simulink model "VDCHyd2020a"  (R2020a)
settings: Solver=daessc  StartTime=0.0  StopTime=simulationEndTime  FixedStep=0.001  RelTol=1e-2
values from neighbouring files (symbols this model uses):
  Bc1_V = [0;0;0;0;0;0]    [initializeSimulationGP.m]
  filtDV = init2ndOrderLowPassFilter(35*2*pi,1,controller.dT)    [initializeLowPassFilters.m]
  filtEnc = init2ndOrderLowPassFilter(35*2*pi,1,controller.dT)    [initializeLowPassFilters.m]
undefined symbols (not defined in the file or in its folder): aux, B11_r_B11Tc1, B11_V, B11_Vr, B11Ftot_r, B12_r_B12Tc2, B12_Rot_Tc2, B12_U_Tc2, B12_V, B12_Vr, B12Ftot_r, B31_r_B31B41, B31_V, B31_Vr, B31FTot_r, B32_r_B32B42, B32_Rot_B42, B32_U_B42, B32_V, B32_Vr, B32FTot_r, B41_r_B41Tc1, B41_V, B41_Vr, B41FTot_r, B42_r_B42Tc2, B42_Rot_Tc2, B42_U_Tc2, B42_V, B42_Vr, B42FTot_r, B52_r_B52P32, B52_Rot_P32, B52_U_P32, B52_V, B52_Vr, B52Ftot_r, Bc1_r_Bc1B11, Bc1_r_Bc1B31, Bc1_Vr, Bc1FTot_r, Bc2_r_Bc2B12, Bc2_r_Bc2B32, Bc2_Rot_B12, Bc2_Rot_B32, Bc2_U_B12, Bc2_U_B32, Bc2_V, Bc2_Vr, Bc2Tot_r, controller, cyl1, cyl2, cylT2, D22_V, D22_Vr, D22Fr, DiscIntNeverNeededParam, dq1, dq11 ... (+125)
libraries: sm_lib x34, nesl_utility x15, simulink x11, dspinverses x1
(part 3 of 12)

== system VDCHyd2020a/sbHydraulicManipulatorSimscape/sbTilitLink ==
  P22p_to_P22 : sm_lib/Frames and Transforms/Rigid Transform  TranslationMethod=StandardAxis  TranslationStandardOffset=17  TranslationLengthUnit=mm  TranslationStandardAxis=+Z  TranslationCartesianOffset=[0 0 0]  TranslationROffset=0  TranslationROffsetUnits=m  TranslationZOffset=0  TranslationZOffsetUnits=m  TranslationThetaOffset=0  TranslationThetaOffsetUnits=deg  RotationMethod=None  RotationAngleUnits=deg  RotationStandardAxis=+Z  RotationAngle=0.0  RotationArbitraryAxis=[0 0 1]  FollAlignAxisA=+X  BaseAlignAxisA=+Y  FollAlignAxisB=+Y  BaseAlignAxisB=+Z  RotationSequenceAxes=FollowerAxes  RotationSequence=XYX  RotationSequenceAngles=[0 0 0]  RotationSequenceAnglesUnits=deg  RotationMatrix=[1 0 0; 0 1 0; 0 0 1]
  TiltLinkSolid : sm_lib/Body Elements/File Solid  ExtGeomFileName=07_TiltLinkGP.STEP  UnitType=Custom  ExtGeomFileUnits=m  StepReaderType=OCC  ExportConvexHullGeometry=off  InertiaType=Custom  Mass=33.92850233  MassUnits=kg  CenterOfMass=[0.53783811 -0.04670816 0.00002484]  CenterOfMassUnits=m  MomentsOfInertia=[0.31079192 7.19217974 7.40915161]  MomentsOfInertiaUnits=kg*m^2  ProductsOfInertia=[-0.00058487 0.00275052 -0.58280922]  ProductsOfInertiaUnits=kg*m^2  BasedOnType=Density  Density=7300  DensityUnits=kg/m^3  DoExposeReferenceFrame=off  SerializedFrames=<Frames><Frame><Id>Frame1</Id><Value><Name>F5rot</Name><Origin><Source>GeometricFeature</Source><FeatureName>cylindrical surface 12</FeatureName></Origin><PrimaryAxis><DefinedDirection>+Z</DefinedDirection><Source>ReferenceFrame</Source><SourceDirection>+Z</SourceDirection><FeatureName></FeatureName></PrimaryAxis><SecondaryAxis><DefinedDirection>+X</DefinedDirection><Source>ReferenceFrame</Source><SourceDirection>+X</SourceDirection><FeatureName></FeatureName></SecondaryAxis></Value></Frame><Frame><Id>Frame2</Id><Value><Name>F6</Name><Origin><Source>GeometricFeature</Source><FeatureName>cylindrical surface 13</FeatureName></Origin><PrimaryAxis><DefinedDirection>+Z</DefinedDirection><Source>ReferenceFrame</Source><SourceDirection>+Z</SourceDirection><FeatureName></FeatureName></PrimaryAxis><SecondaryAxis><DefinedDirection>+X</DefinedDirection><Source>ReferenceFrame</Source><SourceDirection>+X</SourceDirection><FeatureName></FeatureName></SecondaryAxis></Value></Frame><Frame><Id>Frame3</Id><Value><Name>P22p</Name><Origin><Source>GeometricFeature</Source><FeatureName>circular curve 59</FeatureName></Origin><PrimaryAxis><DefinedDirection>+Y</DefinedDirection><Source>GeometricFeature</Source><SourceDirection>+Z</SourceDirection><FeatureName>segment 349</FeatureName></PrimaryAxis><SecondaryAxis><DefinedDirection>+X</DefinedDirection><Source>ReferenceFrame</Source><SourceDirection>+X</SourceDirection><FeatureName></FeatureName></SecondaryAxis></Value></Frame><Frame><Id>Frame4</Id><Value><Name>Tc2p</Name><Origin><Source>GeometricFeature</Source><FeatureName>cylindrical surface 13</FeatureName></Origin><PrimaryAxis><DefinedDirection>+X</DefinedDirection><Source>GeometricFeature</Source><SourceDirection>+Z</SourceDirection><FeatureName>segment 205</FeatureName></PrimaryAxis><SecondaryAxis><DefinedDirection>+Y</DefinedDirection><Source>ReferenceFrame</Source><SourceDirection>+X</SourceDirection><FeatureName></FeatureName></SecondaryAxis></Value></Frame><Frame><Id>Frame5</Id><Value><Name>B12</Name><Origin><Source>GeometricFeature</Source><FeatureName>cylindrical surface 12</FeatureName></Origin><PrimaryAxis><DefinedDirection>-X</DefinedDirection><Source>GeometricFeature</Source><SourceDirection>+Z</SourceDirection><FeatureName>segment 203</FeatureName></PrimaryAxis><SecondaryAxis><DefinedDirection>+Y</DefinedDirection><Source>ReferenceFrame</Source><SourceDirection>+X</SourceDirection><FeatureName></FeatureName></SecondaryAxis></Value></Frame></Frames>  GraphicType=FromGeometry  MarkerShape=Sphere  MarkerSize=10  GraphicVisPropType=SimpleVisualProperties  GraphicDiffuseColor=[134 134 255]/255  GraphicSpecularColor=[0.5 0.5 0.5 1.0]  GraphicAmbientColor=[0.15 0.15 0.15 1.0]  GraphicEmissiveColor=[0.0 0.0 0.0 1.0]  GraphicShininess=75  GraphicOpacity=1.0
  P22 : PMIOPort  Side=Left
  Tc2 : PMIOPort  Port=2  Side=Left
  B12 : PMIOPort  Port=3  Side=Left
  F6 : PMIOPort  Port=4  Side=Left
  F5_rot : PMIOPort  Port=5  Side=Right
  connections:
  F5_rot/RConn1 -- TiltLinkSolid/LConn1
  F6/RConn1 -- TiltLinkSolid/RConn1
  P22p_to_P22/RConn1 -- P22/RConn1
  P22p_to_P22/LConn1 -- TiltLinkSolid/LConn2
  Tc2/RConn1 -- TiltLinkSolid/RConn2
  B12/RConn1 -- TiltLinkSolid/LConn3

== system VDCHyd2020a/sbHydraulicManipulatorSimscape/sbTiltCylinderAndTiltPiston ==
  note: Friction force...
  fp2 : Inport
  B32Aux : sm_lib/Frames and Transforms/Rigid Transform  TranslationMethod=None  TranslationStandardOffset=0  TranslationLengthUnit=m  TranslationStandardAxis=+Z  TranslationCartesianOffset=[0 0 0]  TranslationROffset=0  TranslationROffsetUnits=m  TranslationZOffset=0  TranslationZOffsetUnits=m  TranslationThetaOffset=0  TranslationThetaOffsetUnits=deg  RotationMethod=StandardAxis  RotationAngleUnits=deg  RotationStandardAxis=+Y  RotationAngle=90  RotationArbitraryAxis=[0 0 1]  FollAlignAxisA=+X  BaseAlignAxisA=+Y  FollAlignAxisB=+Y  BaseAlignAxisB=+Z  RotationSequenceAxes=FollowerAxes  RotationSequence=XYX  RotationSequenceAngles=[0 0 0]  RotationSequenceAnglesUnits=deg  RotationMatrix=[1 0 0; 0 1 0; 0 0 1]
  B42Aux : sm_lib/Frames and Transforms/Rigid Transform  TranslationMethod=None  TranslationStandardOffset=0  TranslationLengthUnit=m  TranslationStandardAxis=+Z  TranslationCartesianOffset=[0 0 0]  TranslationROffset=0  TranslationROffsetUnits=m  TranslationZOffset=0  TranslationZOffsetUnits=m  TranslationThetaOffset=0  TranslationThetaOffsetUnits=deg  RotationMethod=StandardAxis  RotationAngleUnits=deg  RotationStandardAxis=+Y  RotationAngle=-90  RotationArbitraryAxis=[0 0 1]  FollAlignAxisA=+X  BaseAlignAxisA=+Y  FollAlignAxisB=+Y  BaseAlignAxisB=+Z  RotationSequenceAxes=FollowerAxes  RotationSequence=XYX  RotationSequenceAngles=[0 0 0]  RotationSequenceAnglesUnits=deg  RotationMatrix=[1 0 0; 0 1 0; 0 0 1]
  Constant : Constant  Value=settings.actuatorFrictionON
  Constant1 : Constant  Value=0
  PS-Sim1 : nesl_utility/PS-Simulink Converter  PhysicalDomain=network_engine_domain  SubClassName=ps_output  LeftPortType=input  RightPortType=output  PseudoPeriodic=off  Frequencies=[]  VectorFormat=1-D array  Unit=inherit  AffineConversion=off
      settings: SourceProductBaseCode=SS,PW,VE
  PS-Sim2 : nesl_utility/PS-Simulink Converter  PhysicalDomain=network_engine_domain  SubClassName=ps_output  LeftPortType=input  RightPortType=output  PseudoPeriodic=off  Frequencies=[]  VectorFormat=1-D array  Unit=inherit  AffineConversion=off
      settings: SourceProductBaseCode=SS,PW,VE
  Simulink-PS Converter : nesl_utility/Simulink-PS Converter  PhysicalDomain=network_engine_domain  SubClassName=ps_input  LeftPortType=input  RightPortType=output  PseudoPeriodic=off  Frequencies=[]  NoiseDistribution=none  NoiseParameters=[]  Unit=1  AffineConversion=off  FilteringAndDerivatives=provide  SimscapeFilterOrder=1  InputFilterTimeConstant=0.001  UdotUserProvided=0
      settings: SourceProductBaseCode=SS,PW,VE
  Sum : Sum  Inputs=|+-
  Switch : Switch  Criteria=u2 > Threshold
  TiltCylinderSolid : sm_lib/Body Elements/File Solid  ExtGeomFileName=05_TiltCylGP.STEP  UnitType=FromFile  ExtGeomFileUnits=m  StepReaderType=OCC  ExportConvexHullGeometry=off  InertiaType=Custom  Mass=17.36281648  MassUnits=kg  CenterOfMass=[0 0.31781210 0]  CenterOfMassUnits=m  MomentsOfInertia=[0.90735702 0.03150902 0.90763033]  MomentsOfInertiaUnits=kg*m^2  ProductsOfInertia=[0 0 0]  ProductsOfInertiaUnits=kg*m^2  BasedOnType=Density  Density=7300  DensityUnits=kg/m^3  DoExposeReferenceFrame=off  SerializedFrames=<Frames><Frame><Id>Frame1</Id><Value><Name>B32</Name><Origin><Source>GeometricFeature</Source><FeatureName>cylindrical surface 11</FeatureName></Origin><PrimaryAxis><DefinedDirection>+X</DefinedDirection><Source>ReferenceFrame</Source><SourceDirection>+Y</SourceDirection><FeatureName></FeatureName></PrimaryAxis><SecondaryAxis><DefinedDirection>+Y</DefinedDirection><Source>ReferenceFrame</Source><SourceDirection>-X</SourceDirection><FeatureName></FeatureName></SecondaryAxis></Value></Frame><Frame><Id>Frame2</Id><Value><Name>B32Aux</Name><Origin><Source>GeometricFeature</Source><FeatureName>planar surface 4</FeatureName></Origin><PrimaryAxis><DefinedDirection>+X</DefinedDirection><Source>ReferenceFrame</Source><SourceDirection>+Y</SourceDirection><FeatureName></FeatureName></PrimaryAxis><SecondaryAxis><DefinedDirection>+Y</DefinedDirection><Source>ReferenceFrame</Source><SourceDirection>-X</SourceDirection><FeatureName></FeatureName></SecondaryAxis></Value></Frame></Frames>  GraphicType=FromGeometry  MarkerShape=Sphere  MarkerSize=10  GraphicVisPropType=SimpleVisualProperties  GraphicDiffuseColor=[1 1 119]/255  GraphicSpecularColor=[0.5 0.5 0.5 1.0]  GraphicAmbientColor=[0.15 0.15 0.15 1.0]  GraphicEmissiveColor=[0.0 0.0 0.0 1.0]  GraphicShininess=75  GraphicOpacity=1.0
  TiltPistonSolid : sm_lib/Body Elements/File Solid  ExtGeomFileName=06_TiltPistGP.STEP  UnitType=FromFile  ExtGeomFileUnits=m  StepReaderType=OCC  ExportConvexHullGeometry=off  InertiaType=Custom  Mass=10.34519231  MassUnits=kg  CenterOfMass=[0 0.32981882 0]  CenterOfMassUnits=m  MomentsOfInertia=[0.55759812 0.00370720 0.55785997]  MomentsOfInertiaUnits=kg*m^2  ProductsOfInertia=[0 0 0]  ProductsOfInertiaUnits=kg*m^2  BasedOnType=Density  Density=7850  DensityUnits=kg/m^3  DoExposeReferenceFrame=off  SerializedFrames=<Frames><Frame><Id>Frame2</Id><Value><Name>B42</Name><Origin><Source>GeometricFeature</Source><FeatureName>planar surface 2</FeatureName></Origin><PrimaryAxis><DefinedDirection>+X</DefinedDirection><Source>ReferenceFrame</Source><SourceDirection>+Y</SourceDirection><FeatureName></FeatureName></PrimaryAxis><SecondaryAxis><DefinedDirection>+Y</DefinedDirection><Source>ReferenceFrame</Source><SourceDirection>-X</SourceDirection><FeatureName></FeatureName></SecondaryAxis></Value></Frame><Frame><Id>Frame3</Id><Value><Name>P11</Name><Origin><Source>GeometricFeature</Source><FeatureName>cylindrical surface 8</FeatureName></Origin><PrimaryAxis><DefinedDirection>+X</DefinedDirection><Source>ReferenceFrame</Source><SourceDirection>+Y</SourceDirection><FeatureName></FeatureName></PrimaryAxis><SecondaryAxis><DefinedDirection>+Y</DefinedDirection><Source>ReferenceFrame</Source><SourceDirection>-X</SourceDirection><FeatureName></FeatureName></SecondaryAxis></Value></Frame></Frames>  GraphicType=FromGeometry  MarkerShape=Sphere  MarkerSize=10  GraphicVisPropType=SimpleVisualProperties  GraphicDiffuseColor=[9 232 232]/255  GraphicSpecularColor=[0.5 0.5 0.5 1.0]  GraphicAmbientColor=[0.15 0.15 0.15 1.0]  GraphicEmissiveColor=[0.0 0.0 0.0 1.0]  GraphicShininess=75  GraphicOpacity=1.0
  q21Rotation : sm_lib/Joints/Revolute Joint  JointMode=Normal  SenseConstraintForce=off  SenseConstraintForceX=off  SenseConstraintForceY=off  SenseConstraintForceZ=off  SenseConstraintTorque=off  SenseConstraintTorqueX=off  SenseConstraintTorqueY=off  SenseConstraintTorqueZ=off  SenseTotalForce=off  SenseTotalForceX=off  SenseTotalForceY=off  SenseTotalForceZ=off  SenseTotalTorque=off  SenseTotalTorqueX=off  SenseTotalTorqueY=off  SenseTotalTorqueZ=off  CompositeWrenchDir=FollowerOnBase  CompositeWrenchFrame=BaseFrame  EquilibriumPosition=0  EquilibriumPositionUnits=rad  SpringStiffness=0  SpringStiffnessUnits=N*m/rad  DampingCoefficient=revJoint2.damp  DampingCoefficientUnits=N*m/(rad/s)  TorqueActuationMode=NoTorque  MotionActuationMode=ComputedMotion  SensePosition=off  SenseVelocity=off  SenseAcceleration=off  SenseTorqueForce=off  SenseLowerLimitTorqueForce=off  SenseUpperLimitTorqueForce=off  LowerLimitSpecify=off  LowerLimitBound=-90  LowerLimitBoundUnits=deg  LowerLimitStiffness=1e4  LowerLimitStiffnessUnits=N*m/deg  LowerLimitDamping=10  LowerLimitDampingUnits=N*m/(deg/s)  LowerLimitTransitionRegionWidth=0.1  LowerLimitTransitionRegionWidthUnits=deg  UpperLimitSpecify=off  UpperLimitBound=90  UpperLimitBoundUnits=deg  UpperLimitStiffness=1e4  UpperLimitStiffnessUnits=N*m/deg  UpperLimitDamping=10  UpperLimitDampingUnits=N*m/(deg/s)  UpperLimitTransitionRegionWidth=0.1  UpperLimitTransitionRegionWidthUnits=deg  PositionTargetSpecify=off  PositionTargetPriority=High  PositionTargetValue=0  PositionTargetValueUnits=deg  VelocityTargetSpecify=off  VelocityTargetPriority=High  VelocityTargetValue=0  VelocityTargetValueUnits=deg/s
  q22Rotation : sm_lib/Joints/Revolute Joint  JointMode=Normal  SenseConstraintForce=off  SenseConstraintForceX=off  SenseConstraintForceY=off  SenseConstraintForceZ=off  SenseConstraintTorque=off  SenseConstraintTorqueX=off  SenseConstraintTorqueY=off  SenseConstraintTorqueZ=off  SenseTotalForce=off  SenseTotalForceX=off  SenseTotalForceY=off  SenseTotalForceZ=off  SenseTotalTorque=off  SenseTotalTorqueX=off  SenseTotalTorqueY=off  SenseTotalTorqueZ=off  CompositeWrenchDir=FollowerOnBase  CompositeWrenchFrame=BaseFrame  EquilibriumPosition=0  EquilibriumPositionUnits=rad  SpringStiffness=0  SpringStiffnessUnits=N*m/rad  DampingCoefficient=revJoint2.damp  DampingCoefficientUnits=N*m/(rad/s)  TorqueActuationMode=NoTorque  MotionActuationMode=ComputedMotion  SensePosition=off  SenseVelocity=off  SenseAcceleration=off  SenseTorqueForce=off  SenseLowerLimitTorqueForce=off  SenseUpperLimitTorqueForce=off  LowerLimitSpecify=off  LowerLimitBound=-90  LowerLimitBoundUnits=deg  LowerLimitStiffness=1e4  LowerLimitStiffnessUnits=N*m/deg  LowerLimitDamping=10  LowerLimitDampingUnits=N*m/(deg/s)  LowerLimitTransitionRegionWidth=0.1  LowerLimitTransitionRegionWidthUnits=deg  UpperLimitSpecify=off  UpperLimitBound=90  UpperLimitBoundUnits=deg  UpperLimitStiffness=1e4  UpperLimitStiffnessUnits=N*m/deg  UpperLimitDamping=10  UpperLimitDampingUnits=N*m/(deg/s)  UpperLimitTransitionRegionWidth=0.1  UpperLimitTransitionRegionWidthUnits=deg  PositionTargetSpecify=off  PositionTargetPriority=High  PositionTargetValue=0  PositionTargetValueUnits=deg  VelocityTargetSpecify=off  VelocityTargetPriority=High  VelocityTargetValue=0  VelocityTargetValueUnits=deg/s
  sbFrictionForceRS2 : Subsystem
  x2-translation : sm_lib/Joints/Prismatic Joint  JointMode=Normal  SenseConstraintForce=off  SenseConstraintForceX=off  SenseConstraintForceY=off  SenseConstraintForceZ=off  SenseConstraintTorque=off  SenseConstraintTorqueX=off  SenseConstraintTorqueY=off  SenseConstraintTorqueZ=off  SenseTotalForce=off  SenseTotalForceX=off  SenseTotalForceY=off  SenseTotalForceZ=off  SenseTotalTorque=off  SenseTotalTorqueX=off  SenseTotalTorqueY=off  SenseTotalTorqueZ=off  CompositeWrenchDir=FollowerOnBase  CompositeWrenchFrame=FollowerFrame  EquilibriumPosition=0  EquilibriumPositionUnits=m  SpringStiffness=0  SpringStiffnessUnits=N/m  DampingCoefficient=0  DampingCoefficientUnits=N/(m/s)  TorqueActuationMode=InputTorque  MotionActuationMode=ComputedMotion  SensePosition=on  SenseVelocity=on  SenseAcceleration=off  SenseTorqueForce=off  SenseLowerLimitTorqueForce=off  SenseUpperLimitTorqueForce=off  LowerLimitSpecify=on  LowerLimitBound=0  LowerLimitBoundUnits=m  LowerLimitStiffness=1e6  LowerLimitStiffnessUnits=N/m  LowerLimitDamping=1e3  LowerLimitDampingUnits=N/(m/s)  LowerLimitTransitionRegionWidth=1e-4  LowerLimitTransitionRegionWidthUnits=m  UpperLimitSpecify=on  UpperLimitBound=cyl2.sp  UpperLimitBoundUnits=m  UpperLimitStiffness=1e6  UpperLimitStiffnessUnits=N/m  UpperLimitDamping=1e3  UpperLimitDampingUnits=N/(m/s)  UpperLimitTransitionRegionWidth=1e-4  UpperLimitTransitionRegionWidthUnits=m  PositionTargetSpecify=on  PositionTargetPriority=Low  PositionTargetValue=0.3  PositionTargetValueUnits=m  VelocityTargetSpecify=on  VelocityTargetPriority=High  VelocityTargetValue=0  VelocityTargetValueUnits=m/s
  B32 : PMIOPort  Side=Left
  B42 : PMIOPort  Port=2  Side=Left
  F4 : PMIOPort  Port=3  Side=Right
  F6 : PMIOPort  Port=4  Side=Right
  x2 : Outport
  dx2 : Outport  Port=2
  wires:
  PS-Sim2/1 -> x2/1
  fp2/1 -> sbFrictionForceRS2/2(fp2), Sum/1
  Sum/1 -> Simulink-PS Converter/1
  Switch/1 -> Sum/2
  PS-Sim1/1 -> sbFrictionForceRS2/1(dx2), dx2/1
  sbFrictionForceRS2/1(ff2) -> Switch/1
  Constant1/1 -> Switch/3
  Constant/1 -> Switch/2
  connections:
  TiltCylinderSolid/RConn1 -- B32Aux/LConn1
  x2-translation/RConn1 -- B42Aux/LConn1
  q21Rotation/RConn1 -- TiltCylinderSolid/LConn1 -- B32/RConn1
  B42/RConn1 -- TiltPistonSolid/LConn1 -- B42Aux/RConn1
  B32Aux/RConn1 -- x2-translation/LConn1
  q21Rotation/LConn1 -- F4/RConn1
  TiltPistonSolid/RConn1 -- q22Rotation/LConn1
  q22Rotation/RConn1 -- F6/RConn1
  x2-translation/RConn2 -- PS-Sim2/LConn1
  Simulink-PS Converter/RConn1 -- x2-translation/LConn2
  PS-Sim1/LConn1 -- x2-translation/RConn3

== system VDCHyd2020a/sbVDCController/sbAuxiliaryJointAngles ==
  note: For more details on relations in this subsystem, please see the supplementary pdf at:
      | https://se.mathworks.com/matlabcentral/fileexchange/123465-calculating-actuator-forces-on-a-hardware-target
      |
      | In the paper qj angles are assumed known beforehand...
  note: Calculate q1 and q2 from measured Theta1 and Theta2 angles...
  note: Get inputs...
  note: Process data...
  note: Pass to outputs...
  theta1Filt : Inport
  theta2Filt : Inport  Port=2
  q1Angle : MATLAB Function  TreatAsAtomicUnit=on
  q2Angle : MATLAB Function  TreatAsAtomicUnit=on
  q1 : Outport
  q2 : Outport  Port=2
  wires:
  q2Angle/1(q2) -> [q2]  "q2"
  [q2] -> q2/1  "q2"
  [q1] -> q1/1  "q1"
  q1Angle/1(q1) -> [q1]  "q1"
  [theta1Filt] -> q1Angle/1(theta1)  "theta1Filt"
  [theta2Filt] -> q2Angle/1(theta2)  "theta2Filt"
  theta2Filt/1 -> [theta2Filt]  "theta2Filt"
  theta1Filt/1 -> [theta1Filt]  "theta1Filt"

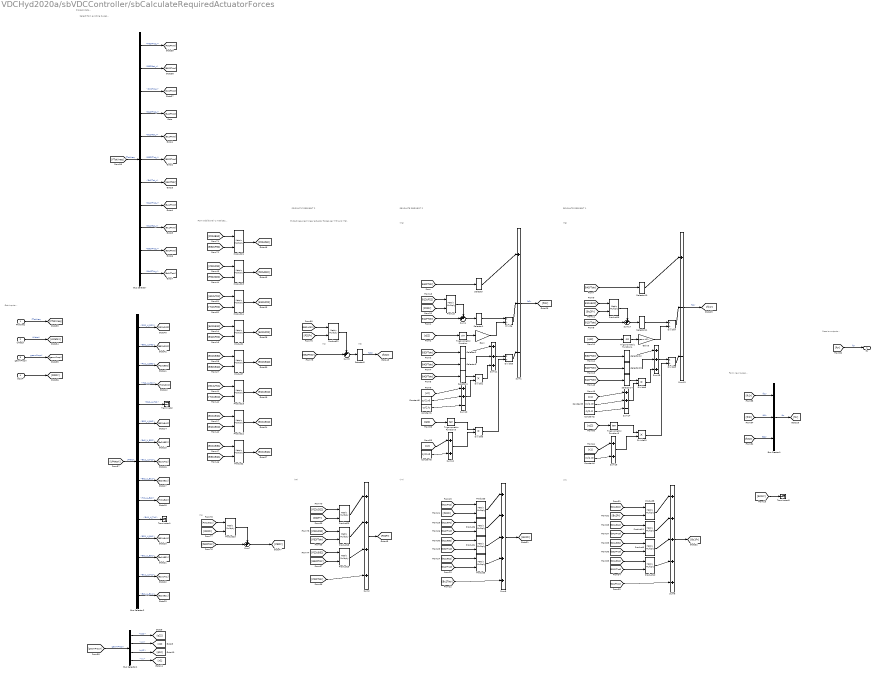
== system VDCHyd2020a/sbVDCController/sbCalculateRequiredActuatorForces ==
  note: (73)
  note: Get inputs...
  note: Select from existing buses...
  note: Form additional U matrices...
  note: (76)
  note: (76)
  note: (77)
  note: (77)
  note: Extract required linear actuator forces per (73) and (76).
  note: Process data...
  note: Form new buses...
  note: Pass to outputs...
  note: (74)
  note: (71)
  note: (72)
  note: REVOLUTE SEGMENT 2
  note: REVOLUTE SEGMENT 1
  note: PRISMATIC SEGMENT 2
  FTotXreq : Inport
  UMatsX : Inport  Port=2
  geomPropX : Inport  Port=3
  D22Fr : Inport  Port=4
  Bus Creator1 : BusCreator  Inputs=fc1r,fc2r,fct2r
  Bus Selector : BusSelector  OutputSignals=FTotPS2req.P32FTot_r,FTotPS2req.B52Ftot_r,FTotPS2req.P22Tot_r,FTotRS2req.B42FTot_r,FTotRS2req.B12Ftot_r,FTotRS2req.B32FTot_r,FTotRS2req.Bc2Tot_r,FTotRS1req.B41FTot_r,FTotRS1req.B11Ftot_r,FTotRS1req.B31FTot_r,FTotRS1req.Bc1FTot_r
  Bus Selector1 : BusSelector  OutputSignals=geomPropRS2.q22,geomPropRS2.x2,geomPropRS1.q12,geomPropRS1.x1
  Bus Selector2 : BusSelector  OutputSignals=UMatsPS2.P32_U_D22,UMatsPS2.B52_U_P32,UMatsPS2.P22_U_B52,UMatsRS2.Tc2_U_P22,UMatsRS2.B42_U_Tc2,UMatsRS2.B32_U_B42,UMatsRS2.Bc2_U_B32,UMatsRS2.B12_U_Tc2,UMatsRS2.Bc2_U_B12,UMatsRS1.Tc1_U_Bc2,UMatsRS1.B41_U_Tc1,UMatsRS1.B31_U_B41,UMatsRS1.Bc1_U_B31,UMatsRS1.B11_U_Tc1,UMatsRS1.Bc1_U_B11
  Constant1 : Constant  Value=cyl2.lc
  Constant2 : Constant  Value=cyl1.lc
  Constant3 : Constant  Value=cyl1.x0
  Constant4 : Constant  Value=cyl1.x0
  Constant5 : Constant  Value=cyl2.x0
  Constant6 : Constant  Value=cyl2.x0
  Divide{,5,7,9} (4 alike) : Product  Inputs=*/
  Divide{1,6,8,10} (4 alike) : Product  Inputs=**
  Gain : Gain  Gain=geom.L21
  Gain5 : Gain  Gain=geom.L11
  Product{,1..16,18..23} (23 alike) : Product  Multiplication=Matrix(*)
  Selector : Selector  IndexMode=Zero-based  InputPortWidth=6  IndexOptions=Index vector (dialog)  Indices=[0]  OutputSizes=1
  Selector{1..3,11..13} (6 alike) : Selector  IndexMode=Zero-based  InputPortWidth=6  IndexOptions=Index vector (dialog)  Indices=[5]  OutputSizes=1
  Selector10 : Selector  IndexMode=Zero-based  InputPortWidth=6  IndexOptions=Index vector (dialog)  Indices=[0]  OutputSizes=1
  Selector14 : Selector  IndexMode=Zero-based  InputPortWidth=6  IndexOptions=Index vector (dialog)  Indices=[1]  OutputSizes=1
  Selector4 : Selector  IndexMode=Zero-based  InputPortWidth=6  IndexOptions=Index vector (dialog)  Indices=[1]  OutputSizes=1
  Selector5 : Selector  IndexMode=Zero-based  InputPortWidth=6  IndexOptions=Index vector (dialog)  Indices=[0]  OutputSizes=1
  Sum1 : Sum  Inputs=|+--
  Sum10 : Sum  Inputs=|++-
  Sum11 : Sum  Inputs=|+++
  Sum12 : Sum  Inputs=|++
  Sum13 : Sum  Inputs=|+--
  Sum14 : Sum  Inputs=|++-
  Sum15 : Sum  Inputs=|+++
  Sum16 : Sum  Inputs=|++
  Sum{3..4,7,17} (4 alike) : Sum  Inputs=++|
  Sum2 : Sum  Inputs=|++++
  Sum5 : Sum  Inputs=|+++++
  Sum6 : Sum  Inputs=|+++++
  Terminator : Terminator
  Terminator1 : Terminator
  Terminator3 : Terminator
  Trigonometric Function : Trigonometry
  Trigonometric Function3 : Trigonometry  Operator=tan
  Trigonometric Function4 : Trigonometry
  Trigonometric Function5 : Trigonometry  Operator=tan
  fcr : Outport
  wires:
  [P22UP32] -> Product13/1
  [P32UD22] -> Product13/2
  Product13/1 -> [P22UD22]
  [Bc1Fr] -> Terminator3/1
  [fct2r] -> Bus Creator1/3  "fct2r"
  Selector5/1 -> [fct2r]  "fct2r"
  Sum3/1 -> Selector5/1
  [B52UP32] -> Product22/1
  [P32Fr] -> Product22/2
  Sum7/1 -> [P32Fr]
  Product23/1 -> Sum7/1
  [P32UD22] -> Product23/1
  [D22Fr] -> Product23/2
  [P32FTotr] -> Sum7/2
  Product22/1 -> Sum3/1
  [B52FTotr] -> Sum3/2
  [P22UB52] -> Product19/1
  [P22UP32] -> Product18/1
  Product21/1 -> [P22UP32]
  [B52UP32] -> Product21/2
  [P22UB52] -> Product21/1
  [P22UD22] -> Product20/1
  [D22Fr] -> Product20/2
  [P32FTotr] -> Product18/2
  [B52FTotr] -> Product19/2
  Product20/1 -> Sum2/1
  Product19/1 -> Sum2/3
  [P22FTotr] -> Sum2/4
  Product18/1 -> Sum2/2
  Sum2/1 -> [P22Fr]
  Bus Selector2/2 -> [B52UP32]  "<B52_U_P32>"
  Bus Selector2/3 -> [P22UB52]  "<P22_U_B52>"
  Bus Selector2/1 -> [P32UD22]  "<P32_U_D22>"
  Bus Selector/1 -> [P32FTotr]  "<P32FTot_r>"
  Bus Selector/2 -> [B52FTotr]  "<B52Ftot_r>"
  Bus Selector/3 -> [P22FTotr]  "<P22Tot_r>"
  [fcr] -> fcr/1  "fcr"
  Bus Creator1/1 -> [fcr]  "fcr"
  [B41FTotr] -> Selector10/1
  Gain5/1 -> Divide7/2
  Trigonometric Function4/1 -> Gain5/1
  Selector10/1 -> Sum13/1
  Divide7/1 -> Sum13/2
  Sum13/1 -> [fc1r]  "fc1r"
  [B11FTotr] -> Sum17/2
  Product16/1 -> Sum17/1
  Sum17/1 -> Selector11/1
  [B11UBc2] -> Product16/1
  [Bc2Fr] -> Product16/2
  Selector11/1 -> Divide7/1
  Divide9/1 -> Sum13/3
  Constant4/1 -> Sum16/2
  [x1] -> Sum16/1
  Selector12/1 -> Sum15/1
  Selector13/1 -> Sum15/2
  Divide8/1 -> Sum15/3
  [B31FTotr] -> Selector12/1
  [B41FTotr] -> Selector13/1
  [B41FTotr] -> Selector14/1
  Selector14/1 -> Divide8/1
  Sum14/1 -> Divide8/2
  Constant2/1 -> Sum14/3
  [x1] -> Sum14/1
  Constant3/1 -> Sum14/2
  [q12] -> Trigonometric Function4/1
  Trigonometric Function5/1 -> Divide10/1
  Sum16/1 -> Divide10/2
  Sum15/1 -> Divide9/1
  Divide10/1 -> Divide9/2
  [q12] -> Trigonometric Function5/1
  [q22] -> Trigonometric Function3/1
  Divide6/1 -> Divide5/2
  Sum11/1 -> Divide5/1
  Sum12/1 -> Divide6/2
  Trigonometric Function3/1 -> Divide6/1
  [geomPropX] -> Bus Selector1/1  "geomPropX"
  [UMatsX] -> Bus Selector2/1  "UMatsX"
  [FTotXreq] -> Bus Selector/1  "FTotXreq"
  D22Fr/1 -> [D22Fr]
  geomPropX/1 -> [geomPropX]  "geomPropX"
  UMatsX/1 -> [UMatsX]  "UMatsX"
  FTotXreq/1 -> [FTotXreq]  "FTotXreq"
  [q22] -> Trigonometric Function/1
  [fc2r] -> Bus Creator1/2  "fc2r"
  [fc1r] -> Bus Creator1/1  "fc1r"
  Constant5/1 -> Sum10/2
  [x2] -> Sum10/1
  Constant1/1 -> Sum10/3
  Sum10/1 -> Divide1/2
  Selector4/1 -> Divide1/1
  [B42FTotr] -> Selector4/1
  [B42FTotr] -> Selector3/1
  [B32FTotr] -> Selector2/1
  Divide1/1 -> Sum11/3
  Selector3/1 -> Sum11/2
  Selector2/1 -> Sum11/1
  [x2] -> Sum12/1
  Constant6/1 -> Sum12/2
  Divide5/1 -> Sum1/3
  Selector1/1 -> Divide/1
  Product12/1 -> [Bc1UBc2]
  [B11UTc1] -> Product15/1
  [Tc1UBc2] -> Product15/2
  Product15/1 -> [B11UBc2]
  [B11UBc2] -> Product12/2
  [Bc1UB11] -> Product12/1
  [Bc2UB12] -> Product1/1
  [B12UP22] -> Product1/2
  Product14/1 -> [B12UP22]
  [Tc2UP22] -> Product14/2
  [B12UTc2] -> Product14/1
  [B31UB41] -> Product2/2
  [Bc1UB31] -> Product2/1
  Product2/1 -> [Bc1UB41]
  Product1/1 -> [Bc2UP22]
  [Bc1UBc2] -> Product8/1
  [Bc2Fr] -> Product8/2
  Product8/1 -> Sum6/1
  [Bc1FTotr] -> Sum6/5
  Product11/1 -> Sum6/2
  Product9/1 -> Sum6/3
  Product10/1 -> Sum6/4
  [B11FTotr] -> Product10/2
  [Bc1UB11] -> Product10/1
  [B31FTotr] -> Product9/2
  [B41FTotr] -> Product11/2
  [Bc1UB41] -> Product11/1
  [Bc1UB31] -> Product9/1
  Sum6/1 -> [Bc1Fr]
  Sum5/1 -> [Bc2Fr]
  [Bc2UB32] -> Product4/1
  [Bc2UB42] -> Product6/1
  Product7/1 -> [Bc2UB42]
  [Bc2UB32] -> Product7/1
  [B32UB42] -> Product7/2
  [B42FTotr] -> Product6/2
  [B32FTotr] -> Product4/2
  [Bc2UB12] -> Product5/1
  [B12FTotr] -> Product5/2
  Product5/1 -> Sum5/4
  Product4/1 -> Sum5/3
  Product6/1 -> Sum5/2
  [Bc2Totr] -> Sum5/5
  Product3/1 -> Sum5/1
  [P22Fr] -> Product3/2
  [P22Fr] -> Product/2
  [Bc2UP22] -> Product3/1
  [B12UP22] -> Product/1
  Sum4/1 -> Selector1/1
  Product/1 -> Sum4/1
  [B12FTotr] -> Sum4/2
  Bus Selector2/15 -> [Bc1UB11]  "<Bc1_U_B11>"
  Bus Selector2/14 -> [B11UTc1]  "<B11_U_Tc1>"
  Bus Selector2/13 -> [Bc1UB31]  "<Bc1_U_B31>"
  Bus Selector2/12 -> [B31UB41]  "<B31_U_B41>"
  Bus Selector2/11 -> Terminator1/1  "<B41_U_Tc1>"
  Bus Selector2/10 -> [Tc1UBc2]  "<Tc1_U_Bc2>"
  Bus Selector2/9 -> [Bc2UB12]  "<Bc2_U_B12>"
  Bus Selector2/8 -> [B12UTc2]  "<B12_U_Tc2>"
  Bus Selector2/7 -> [Bc2UB32]  "<Bc2_U_B32>"
  Bus Selector2/6 -> [B32UB42]  "<B32_U_B42>"
  Bus Selector2/5 -> Terminator/1  "<B42_U_Tc2>"
  Bus Selector2/4 -> [Tc2UP22]  "<Tc2_U_P22>"
  Sum1/1 -> [fc2r]  "fc2r"
  Divide/1 -> Sum1/2
  Selector/1 -> Sum1/1
  Trigonometric Function/1 -> Gain/1
  Gain/1 -> Divide/2
  Bus Selector1/3 -> [q12]  "<q12>"
  Bus Selector1/4 -> [x1]  "<x1>"
  Bus Selector1/2 -> [x2]  "<x2>"
  Bus Selector1/1 -> [q22]  "<q22>"
  [B42FTotr] -> Selector/1
  Bus Selector/11 -> [Bc1FTotr]  "<Bc1FTot_r>"
  Bus Selector/10 -> [B31FTotr]  "<B31FTot_r>"
  Bus Selector/9 -> [B11FTotr]  "<B11Ftot_r>"
  Bus Selector/8 -> [B41FTotr]  "<B41FTot_r>"
  Bus Selector/7 -> [Bc2Totr]  "<Bc2Tot_r>"
  Bus Selector/5 -> [B12FTotr]  "<B12Ftot_r>"
  Bus Selector/6 -> [B32FTotr]  "<B32FTot_r>"
  Bus Selector/4 -> [B42FTotr]  "<B42FTot_r>"

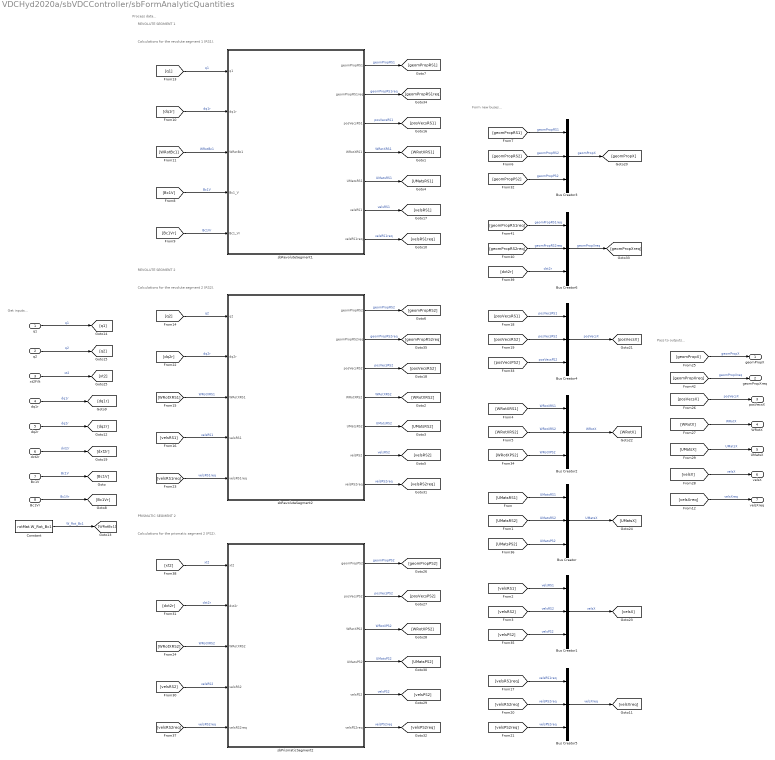
== system VDCHyd2020a/sbVDCController/sbFormAnalyticQuantities ==
  note: Calculations for the prismatic segment 2 (PS2).
  note: Calculations for the revolute segment 2 (RS2).
  note: Calculations for the revolute segment 1 (RS1).
  note: Get inputs...
  note: Process data...
  note: Form new buses...
  note: Pass to outputs...
  note: REVOLUTE SEGMENT 1
  note: REVOLUTE SEGMENT 2
  note: PRISMATIC SEGMENT 2
  q1 : Inport  Unit=rad  PortDimensions=1
  q2 : Inport  Port=2  Unit=rad  PortDimensions=1
  xt2Filt : Inport  Port=3  Unit=m  PortDimensions=1
  dq1r : Inport  Port=4  Unit=rad/s  PortDimensions=1
  dq2r : Inport  Port=5  Unit=rad/s  PortDimensions=1
  dxt2r : Inport  Port=6  Unit=m/s  PortDimensions=1
  Bc1V : Inport  Port=7
  Bc1Vr : Inport  Port=8
  Bus Creator{,2..4} (4 alike) : BusCreator  Inputs=3
  Bus Creator1 : BusCreator  Inputs=velsRS1,velsRS2,velsPS2
  Bus Creator5 : BusCreator  Inputs=velsRS1req,velsRS2req,velsPS2req
  Bus Creator6 : BusCreator  Inputs=geomPropRS1req,geomPropRS2req,dxt2r
  Constant : Constant  Value=rotMat.W_Rot_Bc1
  sbPrismaticSegment2 : Subsystem
      mask Display: image('$imagefile'); % Use "Edit Image" on toolstrip to change.
  sbRevoluteSegment1 : Subsystem
      mask Display: image('$imagefile'); % Use "Edit Image" on toolstrip to change.
  sbRevoluteSegment2 : Subsystem
      mask Display: image('$imagefile'); % Use "Edit Image" on toolstrip to change.
  geomPropX : Outport
  geomPropXreq : Outport  Port=2
  posVecsX : Outport  Port=3
  WRotX : Outport  Port=4
  UMatsX : Outport  Port=5
  velsX : Outport  Port=6
  velsXreq : Outport  Port=7
  wires:
  Bc1V/1 -> [Bc1V]  "Bc1V"
  [velsPS2] -> Bus Creator1/3  "velsPS2"
  [UMatsPS2] -> Bus Creator/3  "UMatsPS2"
  sbPrismaticSegment2/4(UMatsPS2) -> [UMatsPS2]  "UMatsPS2"
  sbPrismaticSegment2/5(velsPS2) -> [velsPS2]  "velsPS2"
  [WRotXPS2] -> Bus Creator2/3  "WRotXPS2"
  sbPrismaticSegment2/3(WRotXPS2) -> [WRotXPS2]  "WRotXPS2"
  [posVecsPS2] -> Bus Creator4/3  "posVecsPS2"
  sbPrismaticSegment2/2(posVecsPS2) -> [posVecsPS2]  "posVecsPS2"
  [geomPropPS2] -> Bus Creator3/3  "geomPropPS2"
  sbPrismaticSegment2/1(geomPropPS2) -> [geomPropPS2]  "geomPropPS2"
  [velsRS2] -> sbPrismaticSegment2/4(velsRS2)  "velsRS2"
  [WRotXRS2] -> sbPrismaticSegment2/3(WRotXRS2)  "WRotXRS2"
  [dxt2r] -> sbPrismaticSegment2/2(dxt2r)  "dxt2r"
  xt2Filt/1 -> [xt2]  "xt2"
  [UMatsX] -> UMatsX/1  "UMatsX"
  [velsX] -> velsX/1  "velsX"
  [WRotX] -> WRotX/1  "WRotX"
  [posVecsX] -> posVecsX/1  "posVecsX"
  [geomPropX] -> geomPropX/1  "geomPropX"
  Bus Creator/1 -> [UMatsX]  "UMatsX"
  Bus Creator1/1 -> [velsX]  "velsX"
  Bus Creator2/1 -> [WRotX]  "WRotX"
  Bus Creator4/1 -> [posVecsX]  "posVecsX"
  Bus Creator3/1 -> [geomPropX]  "geomPropX"
  [geomPropRS1] -> Bus Creator3/1  "geomPropRS1"
  [geomPropRS2] -> Bus Creator3/2  "geomPropRS2"
  [velsRS2] -> Bus Creator1/2  "velsRS2"
  [velsRS1] -> Bus Creator1/1  "velsRS1"
  [UMatsRS1] -> Bus Creator/1  "UMatsRS1"
  [UMatsRS2] -> Bus Creator/2  "UMatsRS2"
  [WRotXRS1] -> Bus Creator2/1  "WRotXRS1"
  [WRotXRS2] -> Bus Creator2/2  "WRotXRS2"
  [posVecsRS2] -> Bus Creator4/2  "posVecsRS2"
  sbRevoluteSegment2/3(posVecsRS2) -> [posVecsRS2]  "posVecsRS2"
  [posVecsRS1] -> Bus Creator4/1  "posVecsRS1"
  sbRevoluteSegment1/3(posVecsRS1) -> [posVecsRS1]  "posVecsRS1"
  [q2] -> sbRevoluteSegment2/1(q2)  "q2"
  q2/1 -> [q2]  "q2"
  [q1] -> sbRevoluteSegment1/1(q1)  "q1"
  q1/1 -> [q1]  "q1"
  [Bc1V] -> sbRevoluteSegment1/4(Bc1_V)  "Bc1V"
  [WRotBc1] -> sbRevoluteSegment1/3(WRotBc1)  "WRotBc1"
  Constant/1 -> [WRotBc1]  "W_Rot_Bc1"
  sbRevoluteSegment1/1(geomPropRS1) -> [geomPropRS1]  "geomPropRS1"
  sbRevoluteSegment2/1(geomPropRS2) -> [geomPropRS2]  "geomPropRS2"
  sbRevoluteSegment2/4(WRotXRS2) -> [WRotXRS2]  "WRotXRS2"
  [WRotXRS1] -> sbRevoluteSegment2/3(WRotXRS1)  "WRotXRS1"
  sbRevoluteSegment1/4(WRotXRS1) -> [WRotXRS1]  "WRotXRS1"
  sbRevoluteSegment1/5(UMatsRS1) -> [UMatsRS1]  "UMatsRS1"
  sbRevoluteSegment2/5(UMatsRS2) -> [UMatsRS2]  "UMatsRS2"
  sbRevoluteSegment2/6(velsRS2) -> [velsRS2]  "velsRS2"
  [velsRS1] -> sbRevoluteSegment2/4(velsRS1)  "velsRS1"
  sbRevoluteSegment1/6(velsRS1) -> [velsRS1]  "velsRS1"
  Bc1Vr/1 -> [Bc1Vr]  "Bc1Vr"
  dq1r/1 -> [dq1r]  "dq1r"
  [dq1r] -> sbRevoluteSegment1/2(dq1r)  "dq1r"
  [Bc1Vr] -> sbRevoluteSegment1/5(Bc1_Vr)  "Bc1Vr"
  sbRevoluteSegment1/7(velsRS1req) -> [velsRS1req]  "velsRS1req"
  [velsXreq] -> velsXreq/1  "velsXreq"
  [velsRS2req] -> Bus Creator5/2  "velsRS2req"
  [velsRS1req] -> Bus Creator5/1  "velsRS1req"
  Bus Creator5/1 -> [velsXreq]  "velsXreq"
  [velsPS2req] -> Bus Creator5/3  "velsPS2req"
  dq2r/1 -> [dq2r]  "dq2r"
  dxt2r/1 -> [dxt2r]  "dxt2r"
  sbRevoluteSegment2/7(velsRS2req) -> [velsRS2req]  "velsRS2req"
  [dq2r] -> sbRevoluteSegment2/2(dq2r)  "dq2r"
  [velsRS1req] -> sbRevoluteSegment2/5(velsRS1req)  "velsRS1req"
  [velsRS2req] -> sbPrismaticSegment2/5(velsRS2req)  "velsRS2req"
  [xt2] -> sbPrismaticSegment2/1(xt2)  "xt2"
  sbPrismaticSegment2/6(velsPS2req) -> [velsPS2req]  "velsPS2req"
  [geomPropRS2req] -> Bus Creator6/2  "geomPropRS2req"
  [geomPropRS1req] -> Bus Creator6/1  "geomPropRS1req"
  Bus Creator6/1 -> [geomPropXreq]  "geomPropXreq"
  [dxt2r] -> Bus Creator6/3  "dxt2r"
  sbRevoluteSegment1/2(geomPropRS1req) -> [geomPropRS1req]  "geomPropRS1req"
  sbRevoluteSegment2/2(geomPropRS2req) -> [geomPropRS2req]  "geomPropRS2req"
  [geomPropXreq] -> geomPropXreq/1  "geomPropXreq"

== system VDCHyd2020a/sbVDCController/sbFormTotalRequiredForces ==
  note: Get inputs...
  note: Pass to outputs...
  note: Form new buses...
  note: Process data...
  velsX : Inport
  velsXreq : Inport  Port=2
  WRotX : Inport  Port=3
  updateActive : Inport  Port=4
  updateReset : Inport  Port=5
  Bus Creator : BusCreator  Inputs=FTotRS1req,FTotRS2req,FTotPS2req
  sbTotalRequiredForcesPS2 : Subsystem
      mask Display: image('$imagefile'); % Use "Edit Image" on toolstrip to change.
  sbTotalRequiredForcesRS1 : Subsystem
      mask Display: image('$imagefile'); % Use "Edit Image" on toolstrip to change.
  sbTotalRequiredForcesRS2 : Subsystem
      mask Display: image('$imagefile'); % Use "Edit Image" on toolstrip to change.
  FTotXreq : Outport
  wires:
  [FTotPS2req] -> Bus Creator/3  "FTotPS2req"
  sbTotalRequiredForcesPS2/1(FTotRS2req) -> [FTotPS2req]  "FTotPS2req"
  [velsX] -> sbTotalRequiredForcesPS2/1(velsX)  "velsX"
  [WRotX] -> sbTotalRequiredForcesPS2/3(WRotX)  "WRotX"
  Bus Creator/1 -> [FTotXreq]  "FTotXreq"
  [FTotXreq] -> FTotXreq/1  "FTotXreq"
  [FTotRS1req] -> Bus Creator/1  "FTotRS1req"
  [FTotRS2req] -> Bus Creator/2  "FTotRS2req"
  sbTotalRequiredForcesRS1/1(FTotRS1req) -> [FTotRS1req]  "FTotRS1req"
  sbTotalRequiredForcesRS2/1(FTotRS2req) -> [FTotRS2req]  "FTotRS2req"
  [WRotX] -> sbTotalRequiredForcesRS2/3(WRotX)  "WRotX"
  [velsX] -> sbTotalRequiredForcesRS2/1(velsX)  "velsX"
  [velsX] -> sbTotalRequiredForcesRS1/1(velsX)  "velsX"
  WRotX/1 -> [WRotX]  "WRotX"
  velsX/1 -> [velsX]  "velsX"
  [velsXreq] -> sbTotalRequiredForcesRS1/2(velsXreq)  "velsXreq"
  [WRotX] -> sbTotalRequiredForcesRS1/3(WRotX)  "WRotX"
  [updateActive] -> sbTotalRequiredForcesRS1/4(updateActive)  "updateActive"
  [updateReset] -> sbTotalRequiredForcesRS1/5(updateReset)  "updateReset"
  velsXreq/1 -> [velsXreq]  "velsXreq"
  [updateActive] -> sbTotalRequiredForcesRS2/4(updateActive)  "updateActive"
  [updateReset] -> sbTotalRequiredForcesRS2/5(updateReset)  "updateReset"
  [velsXreq] -> sbTotalRequiredForcesRS2/2(velsXreq)  "velsXreq"
  updateActive/1 -> [updateActive]  "updateActive"
  updateReset/1 -> [updateReset]  "updateReset"
  [velsXreq] -> sbTotalRequiredForcesPS2/2(velsXreq)  "velsXreq"
  [updateActive] -> sbTotalRequiredForcesPS2/4(updateActive)  "updateActive"
  [updateReset] -> sbTotalRequiredForcesPS2/5(updateReset)  "updateReset"
